simulink subsystem "joint_power"  (R2024b)
settings: Solver=VariableStepAuto  StartTime=0.0  StopTime=10.0  RelTol=1e-3
settings Model: Creator=Mohammed Hany  LastModifiedBy=Mohammed Hany

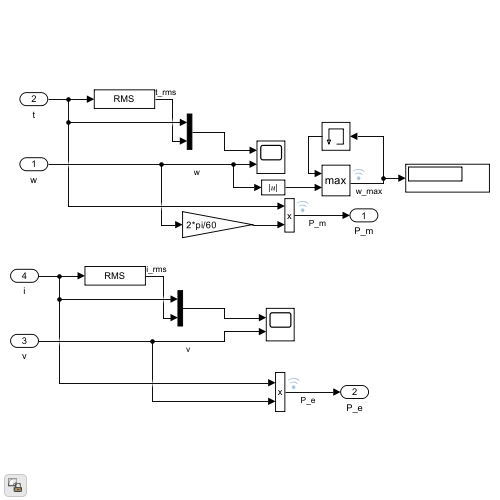
[thumbnail: Simulink's stored preview of the top-level diagram]
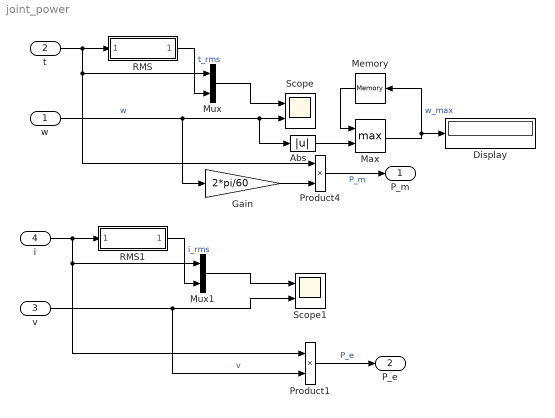
== system joint_power ==
  w : Inport
  t : Inport  Port=2
  v : Inport  Port=3
  i : Inport  Port=4
  Abs : Abs  SaturateOnIntegerOverflow=off
  Display : Display
  Gain : Gain  Gain=2*pi/60
  Max : MinMax  Function=max  Inputs=2
  Memory : Memory
  Mux : Mux  Inputs=2
  Mux1 : Mux  Inputs=2
  Product1 : Product
  Product4 : Product
  RMS : Subsystem  ReferencedSubsystem=RMS
  RMS1 : Subsystem  ReferencedSubsystem=RMS
  Scope : Scope  NumInputPorts=2
  Scope1 : Scope  NumInputPorts=2
  P_m : Outport
  P_e : Outport  Port=2
  wires:
  w/1 -> Scope/2, Abs/1, Gain/1  "w"
  t/1 -> RMS/1, Mux/1, Product4/1
  RMS/1 -> Mux/2  "t_rms"
  Product4/1 -> P_m/1  "P_m"
  Mux/1 -> Scope/1
  i/1 -> RMS1/1, Mux1/1, Product1/1
  v/1 -> Scope1/2, Product1/2  "v"
  Product1/1 -> P_e/1  "P_e"
  RMS1/1 -> Mux1/2  "i_rms"
  Mux1/1 -> Scope1/1
  Gain/1 -> Product4/2
  Max/1 -> Display/1, Memory/1  "w_max"
  Memory/1 -> Max/1
  Abs/1 -> Max/2
